simulink model "Inverter"  (R2016b)
settings: Solver=VariableStepAuto  StartTime=0.0  StopTime=1  RelTol=1e-3
undefined symbols (not defined in the file): Tmli, Vdc
libraries: powerlib x11, simulink x4
settings Model: Creator=21277  LastModifiedBy=21277
settings DataIOCC: ReturnWorkspaceOutputs=on
settings DebuggingCC: UnconnectedInputMsg=none  UnconnectedOutputMsg=none  UnconnectedLineMsg=none  SFMachineParentedDataDiag=error
settings ModelReferenceCC: EnableRefExpFcnMdlSchedulingChecks=off
settings SFSimCC: SimUseLocalCustomCode=on
settings RTWCC: RTWUseLocalCustomCode=on

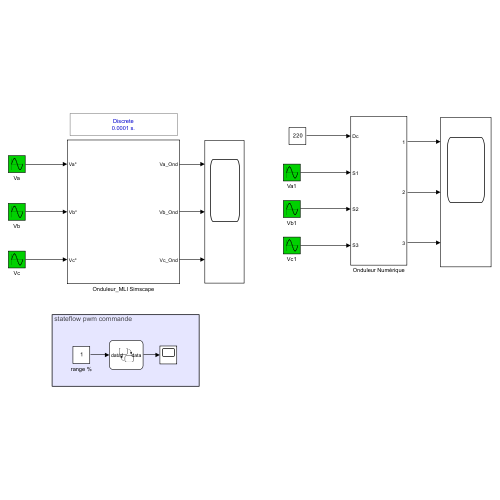
[thumbnail: Simulink's stored preview of the top-level diagram]
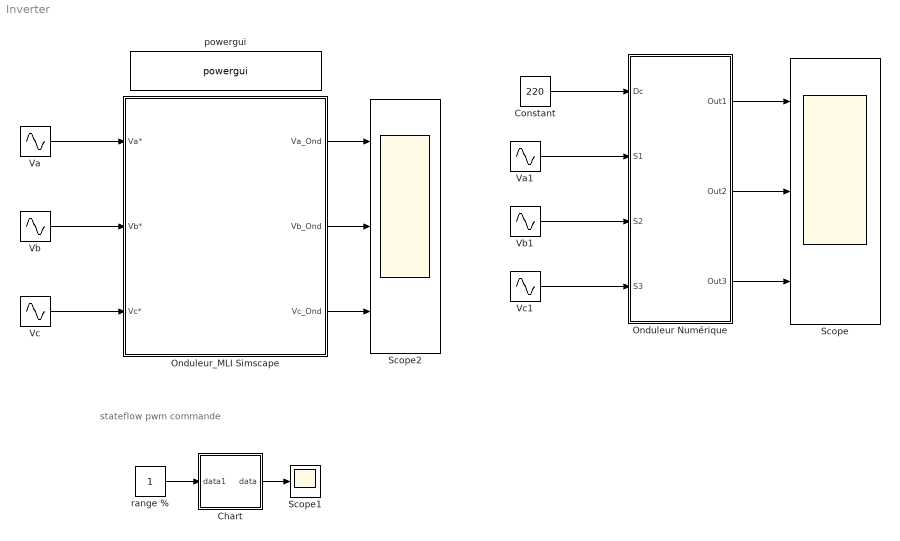
== system Inverter ==
  note: stateflow pwm commande
  Chart : Stateflow chart  TreatAsAtomicUnit=on
  Constant : Constant  Value=220
  Onduleur Numérique : Subsystem
  Onduleur_MLI Simscape : Subsystem
  Scope : Scope  NumInputPorts=3
  Scope1 : Scope
  Scope2 : Scope  NumInputPorts=3
  Va : Sin  Amplitude=100  Frequency=50  SampleTime=0
  Va1 : Sin  Amplitude=100  Frequency=50  SampleTime=0
  Vb : Sin  Amplitude=100  Frequency=50  Phase=2*pi/3  SampleTime=0
  Vb1 : Sin  Amplitude=100  Frequency=50  Phase=2*pi/3  SampleTime=0
  Vc : Sin  Amplitude=100  Frequency=50  Phase=4*pi/3  SampleTime=0
  Vc1 : Sin  Amplitude=100  Frequency=50  Phase=4*pi/3  SampleTime=0
  powergui : powerlib/powergui  Priority=1  SimulationMode=Discrete  SampleTime=1e-4  frequency=60  Iterations=50  frequencyindice=0  Pbase=100e6  ErrMax=1e-4  UnitsV=kV  UnitsW=MW  buscounter=0  FunctionMessages=off  echomessages=off  EnableUseOfTLC=off  CurrentSourceSwitches=off  DisableSnubberDevices=off  DisableRonSwitches=off  DisableVfSwitches=off  DisplayEquations=off  AutomaticDiscreteSolvers=off  SolverType=Tustin/Backward Euler (TBE)  Interpol=off  ExternalGateDelay=off  methode=off  Ts=100  x0status=blocks  SPID=on  SwTol=0  HookPort=off  NonlinearTolerance=1e-4  nMaxIteration=100  ContinueOnMaxIteration=off  RestoreLinks=warning  ResistiveCurrentMeasurement=off  Frange=[0:2:500]  Ylog=off  Xlog=on  ShowGrid=off  save=off  variable=ZData  structure=0  ZoomFFT=off  StartTime=0.0  cycles=1  DisplayStyle=1  fundamental=60  FreqAxis=off  MaxFrequency=1000  frequencyindicesteady=1  RmsSteady=1  display=off
  range % : Constant
  wires:
  Va/1 -> Onduleur_MLI Simscape/1(Va*)
  Vb/1 -> Onduleur_MLI Simscape/2(Vb*)
  Vc/1 -> Onduleur_MLI Simscape/3(Vc*)
  Onduleur_MLI Simscape/2(Vb_Ond) -> Scope2/2
  Onduleur_MLI Simscape/1(Va_Ond) -> Scope2/1
  Onduleur_MLI Simscape/3(Vc_Ond) -> Scope2/3
  Va1/1 -> Onduleur Numérique/2(S1)
  Vb1/1 -> Onduleur Numérique/3(S2)
  Vc1/1 -> Onduleur Numérique/4(S3)
  Onduleur Numérique/3(Out3) -> Scope/3
  Onduleur Numérique/2(Out2) -> Scope/2
  Onduleur Numérique/1(Out1) -> Scope/1
  Constant/1 -> Onduleur Numérique/1("Dc ")
  range %/1 -> Chart/1(data1)
  Chart/1(data) -> Scope1/1

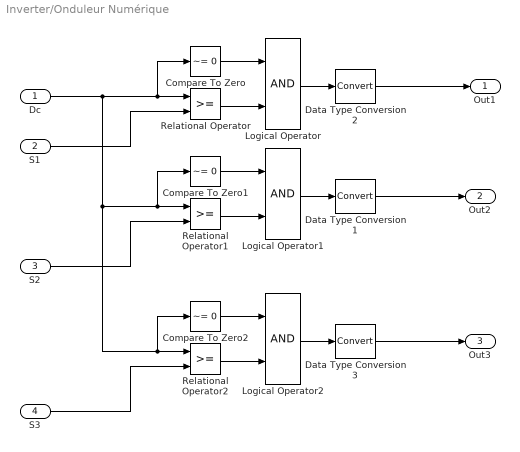
== system Inverter/Onduleur Numérique ==
  "Dc " : Inport
  S1 : Inport  Port=2
  S2 : Inport  Port=3
  S3 : Inport  Port=4
  Compare To Zero : simulink/Logic and Bit Operations/Compare To Zero  relop=~=  OutDataTypeStr=boolean
  Compare To Zero1 : simulink/Logic and Bit Operations/Compare To Zero  relop=~=  OutDataTypeStr=boolean
  Compare To Zero2 : simulink/Logic and Bit Operations/Compare To Zero  relop=~=  OutDataTypeStr=boolean
  Data Type Conversion1 : DataTypeConversion
  Data Type Conversion2 : DataTypeConversion
  Data Type Conversion3 : DataTypeConversion
  Logical Operator : Logic  AllPortsSameDT=off  OutDataTypeStr=boolean
  Logical Operator1 : Logic  AllPortsSameDT=off  OutDataTypeStr=boolean
  Logical Operator2 : Logic  AllPortsSameDT=off  OutDataTypeStr=boolean
  Relational Operator : RelationalOperator  OutDataTypeStr=boolean  RndMeth=Simplest
  Relational Operator1 : RelationalOperator  OutDataTypeStr=boolean  RndMeth=Simplest
  Relational Operator2 : RelationalOperator  OutDataTypeStr=boolean  RndMeth=Simplest
  Out1 : Outport
  Out2 : Outport  Port=2
  Out3 : Outport  Port=3
  wires:
  Data Type Conversion2/1 -> Out1/1
  Logical Operator/1 -> Data Type Conversion2/1
  Compare To Zero/1 -> Logical Operator/1
  Relational Operator/1 -> Logical Operator/2
  S1/1 -> Relational Operator/2
  S2/1 -> Relational Operator1/2
  Relational Operator1/1 -> Logical Operator1/2
  Compare To Zero1/1 -> Logical Operator1/1
  Logical Operator1/1 -> Data Type Conversion1/1
  Data Type Conversion1/1 -> Out2/1
  Data Type Conversion3/1 -> Out3/1
  Logical Operator2/1 -> Data Type Conversion3/1
  Compare To Zero2/1 -> Logical Operator2/1
  Relational Operator2/1 -> Logical Operator2/2
  "Dc "/1 -> Relational Operator2/1, Compare To Zero2/1, Compare To Zero1/1, Relational Operator1/1, Relational Operator/1, Compare To Zero/1
  S3/1 -> Relational Operator2/2

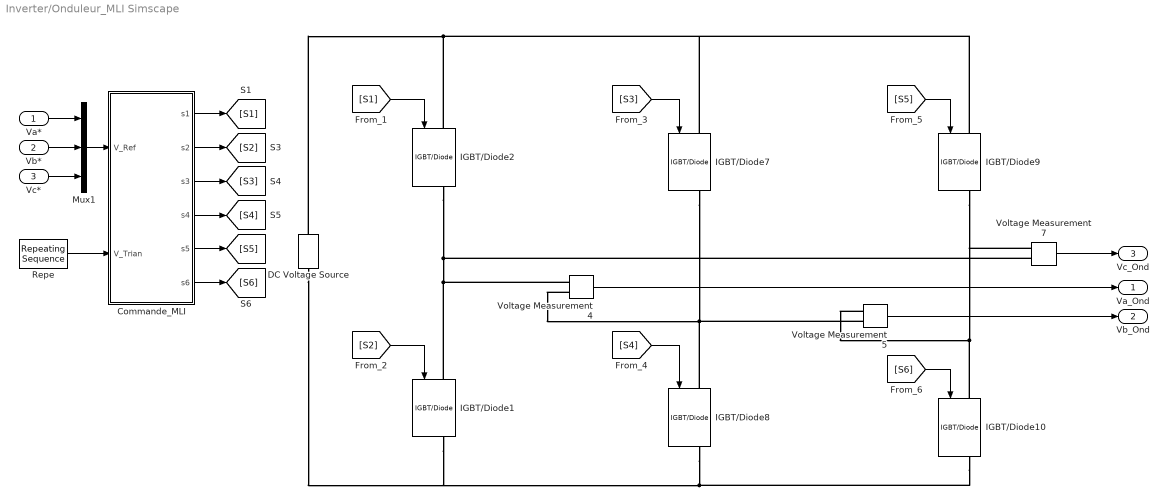
== system Inverter/Onduleur_MLI Simscape ==
  Va* : Inport
  Vb* : Inport  Port=2
  Vc* : Inport  Port=3
  Commande_MLI : Subsystem
  DC Voltage Source : powerlib/Electrical Sources/DC Voltage Source  Amplitude=100  Measurements=None
  IGBT/Diode{1..2,7..10} (6 alike) : powerlib/Power Electronics/IGBT//Diode  Ron=1e-3  Rs=1e5  Cs=inf  Measurements=on
  Mux1 : Mux  Inputs=3
  Repe : simulink/Sources/Repeating Sequence  rep_seq_t=[0 0.5 1]*Tmli  rep_seq_y=[-1 1 -1]*Vdc
  Voltage Measurement4 : powerlib/Measurements/Voltage Measurement  PhasorSimulation=off  OutputType=Complex  PSBequivalent=0
  Voltage Measurement5 : powerlib/Measurements/Voltage Measurement  PhasorSimulation=off  OutputType=Complex  PSBequivalent=0
  Voltage Measurement7 : powerlib/Measurements/Voltage Measurement  PhasorSimulation=off  OutputType=Complex  PSBequivalent=0
  Va_Ond : Outport
  Vb_Ond : Outport  Port=2
  Vc_Ond : Outport  Port=3
  wires:
  Voltage Measurement4/1 -> Va_Ond/1
  Voltage Measurement7/1 -> Vc_Ond/1
  Voltage Measurement5/1 -> Vb_Ond/1
  [S4] -> IGBT/Diode8/1
  Va*/1 -> Mux1/1
  [S5] -> IGBT/Diode9/1
  [S6] -> IGBT/Diode10/1
  Commande_MLI/3(s3) -> [S3]
  Commande_MLI/5(s5) -> [S5]
  [S3] -> IGBT/Diode7/1
  Vc*/1 -> Mux1/3
  Commande_MLI/2(s2) -> [S2]
  [S2] -> IGBT/Diode1/1
  Vb*/1 -> Mux1/2
  Commande_MLI/1(s1) -> [S1]
  [S1] -> IGBT/Diode2/1
  Mux1/1 -> Commande_MLI/1(V_Ref)
  Commande_MLI/6(s6) -> [S6]
  Repe/1 -> Commande_MLI/2(V_Trian)
  Commande_MLI/4(s4) -> [S4]
  connections:
  IGBT/Diode8/LConn1 -- Voltage Measurement4/LConn2 -- Voltage Measurement5/LConn1 -- IGBT/Diode7/RConn1
  IGBT/Diode2/LConn1 -- DC Voltage Source/RConn1 -- IGBT/Diode7/LConn1 -- IGBT/Diode9/LConn1
  IGBT/Diode10/RConn1 -- IGBT/Diode8/RConn1 -- DC Voltage Source/LConn1 -- IGBT/Diode1/RConn1
  IGBT/Diode10/LConn1 -- IGBT/Diode9/RConn1 -- Voltage Measurement7/LConn1 -- Voltage Measurement5/LConn2
  IGBT/Diode2/RConn1 -- Voltage Measurement7/LConn2 -- IGBT/Diode1/LConn1 -- Voltage Measurement4/LConn1

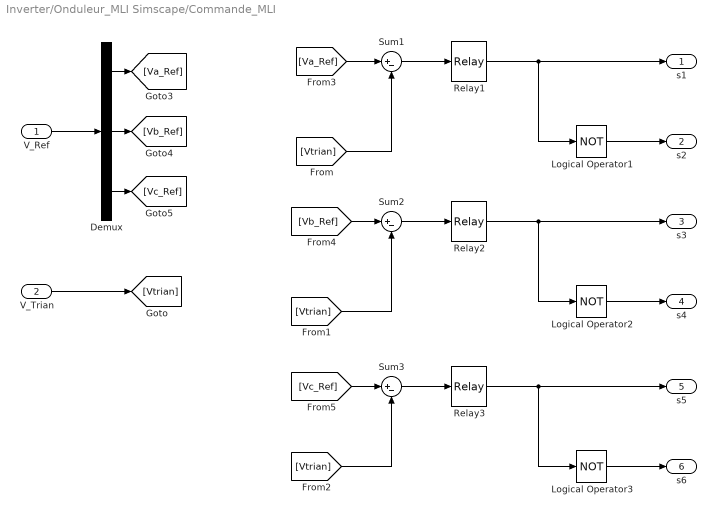
== system Inverter/Onduleur_MLI Simscape/Commande_MLI ==
  V_Ref : Inport
  V_Trian : Inport  Port=2
  Demux : Demux  Outputs=3
  Logical Operator1 : Logic  Operator=NOT  AllPortsSameDT=off  OutDataTypeStr=boolean
  Logical Operator2 : Logic  Operator=NOT  AllPortsSameDT=off  OutDataTypeStr=boolean
  Logical Operator3 : Logic  Operator=NOT  AllPortsSameDT=off  OutDataTypeStr=boolean
  Relay1 : Relay  OffSwitchValue=-eps
  Relay2 : Relay  OffSwitchValue=-eps
  Relay3 : Relay  OffSwitchValue=-eps
  Sum1 : Sum  Inputs=|+-
  Sum2 : Sum  Inputs=|+-
  Sum3 : Sum  Inputs=|+-
  s1 : Outport
  s2 : Outport  Port=2
  s3 : Outport  Port=3
  s4 : Outport  Port=4
  s5 : Outport  Port=5
  s6 : Outport  Port=6
  wires:
  Logical Operator2/1 -> s4/1
  Relay2/1 -> s3/1, Logical Operator2/1
  Sum2/1 -> Relay2/1
  V_Ref/1 -> Demux/1
  Relay1/1 -> s1/1, Logical Operator1/1
  Logical Operator1/1 -> s2/1
  Sum1/1 -> Relay1/1
  Sum3/1 -> Relay3/1
  Logical Operator3/1 -> s6/1
  Relay3/1 -> s5/1, Logical Operator3/1
  [Vtrian] -> Sum1/2
  [Vtrian] -> Sum2/2
  [Vtrian] -> Sum3/2
  [Va_Ref] -> Sum1/1
  [Vb_Ref] -> Sum2/1
  [Vc_Ref] -> Sum3/1
  Demux/1 -> [Va_Ref]
  Demux/2 -> [Vb_Ref]
  Demux/3 -> [Vc_Ref]
  V_Trian/1 -> [Vtrian]

== stateflow chart Inverter/Chart ==
  state N1
    entry:
    out=1;
    i=1;
    during:
    i=i+1;
  state N2
    entry:
    out=0;
    during:
    i=i+1;
  (default) -> N1
  N1 -> N2 : [i>=in]
  N2 -> N1 : [i>=99]
  data: data2 local double; data1 input double; data output double
